simulink model "Kursovoy"  (Simulink 8.6)
settings: Solver=ode45  StartTime=0.0  StopTime=10  MaxStep=10e-6  RelTol=1e-3
values from neighbouring files (symbols this model uses):
  h_r = 0.9    [Drive1.m]    (also in Drive2.m; Drive3.m)
  i_r = 282.65    [Drive1.m]    (also in Drive2.m = 749.309; Drive3.m = 758.23)
  k_m = 0.704    [Drive1.m]    (also in Drive2.m = 0.694; Drive3.m = 0.744)
  k_p = 1.451E+4    (= 14510)    [Drive1.m]    (also in Drive2.m = 1621; Drive3.m = 1214)
  k_s = 6.41E+9    (= 6410000000)    [Drive1.m]    (also in Drive2.m = 1179000000; Drive3.m = 900400000)
  k_t = 1.787    [Drive1.m]    (also in Drive2.m = 1.208; Drive3.m = 3.846)
  Mdist_max = 1.326E+3    (= 1326)    [Drive1.m]    (also in Drive2.m = 15020; Drive3.m = 5965)
  Q_s = 0.991    [Drive1.m]    (also in Drive2.m = 0.412; Drive3.m = 0.252)
  T = 3.333E-6    (= 3.333e-06)    [Drive1.m]    (also in Drive2.m; Drive3.m)
  T1 = 0.219    [Drive1.m]    (also in Drive2.m = 0.415; Drive3.m = 0.289)
  T2 = 0.053    [Drive1.m]    (also in Drive2.m = 0.093; Drive3.m = 0.077)
  T5 = 7.559E-6    (= 7.559e-06)    [Drive1.m]    (also in Drive2.m = 1.323e-05; Drive3.m = 1.098e-05)
  Tau = 8.22E-4    (= 0.000822)    [Drive1.m]    (also in Drive2.m = 0.001429; Drive3.m = 0.001182)
  Te = 5.977E-3    (= 0.005977)    [Drive1.m]    (also in Drive2.m = 0.006546; Drive3.m = 0.004407)
  Tm = 0.098    [Drive1.m]    (also in Drive2.m = 0.03; Drive3.m = 0.025)
  w_max = 1.112    [Drive1.m]    (also in Drive2.m = 0.419; Drive3.m = 0.414)
  w_s = 1.122    [Drive1.m]    (also in Drive2.m = 1.017; Drive3.m = 1.646)
libraries: simulink x1
settings Model: Creator=divaise  LastModifiedBy=Admin
settings DebuggingCC: FcnCallInpInsideContextMsg=UseLocalSettings

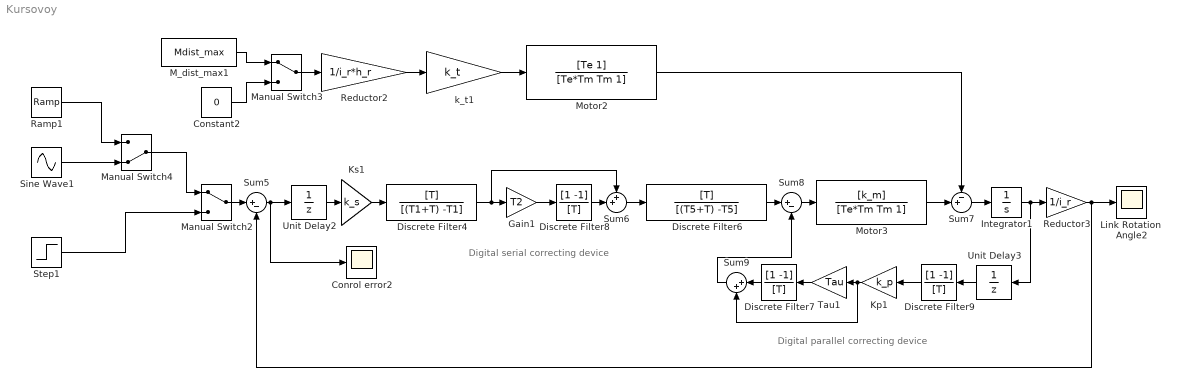
== system Kursovoy ==
  note: Digital serial correcting device
  note: Digital parallel correcting device
  Conrol error2 : Scope
  Constant2 : Constant  Value=0
  Discrete Filter4 : DiscreteFilter  Numerator=[T]  Denominator=[(T1+T) -T1]  SampleTime=T
  Discrete Filter6 : DiscreteFilter  Numerator=[T]  Denominator=[(T5+T) -T5]  SampleTime=T
  Discrete Filter7 : DiscreteFilter  Numerator=[1 -1]  Denominator=[T]  SampleTime=T
  Discrete Filter8 : DiscreteFilter  Numerator=[1 -1]  Denominator=[T]  SampleTime=T
  Discrete Filter9 : DiscreteFilter  Numerator=[1 -1]  Denominator=[T]  SampleTime=T
  Gain1 : Gain  Gain=T2
  Integrator1 : Integrator
  Kp1 : Gain  Gain=k_p
  Ks1 : Gain  Gain=k_s
  Link Rotation  Angle2 : Scope
  M_dist_max1 : Constant  Value=Mdist_max
  Manual Switch2 : ManualSwitch
  Manual Switch3 : ManualSwitch
  Manual Switch4 : ManualSwitch  CurrentSetting=0
  Motor2 : TransferFcn  Numerator=[Te 1]  Denominator=[Te*Tm Tm 1]
  Motor3 : TransferFcn  Numerator=[k_m]  Denominator=[Te*Tm Tm 1]
  Ramp1 : simulink/Sources/Ramp  slope=w_max  start=0  X0=0
  Reductor2 : Gain  Gain=1/i_r*h_r
  Reductor3 : Gain  Gain=1/i_r
  Sine Wave1 : Sin  Amplitude=Q_s  Frequency=w_s  SampleTime=0
  Step1 : Step  Time=0  SampleTime=0
  Sum5 : Sum  Inputs=|+-
  Sum6 : Sum  Inputs=++|
  Sum7 : Sum  Inputs=-+|
  Sum8 : Sum  Inputs=|+-
  Sum9 : Sum  Inputs=|++
  Tau1 : Gain  Gain=Tau
  Unit Delay2 : UnitDelay  SampleTime=T
  Unit Delay3 : UnitDelay  SampleTime=T
  k_t1 : Gain  Gain=k_t
  wires:
  Ramp1/1 -> Manual Switch4/1
  Sine Wave1/1 -> Manual Switch4/2
  Step1/1 -> Manual Switch2/2
  Manual Switch2/1 -> Sum5/1
  Reductor2/1 -> k_t1/1
  k_t1/1 -> Motor2/1
  Sum6/1 -> Discrete Filter6/1
  Motor3/1 -> Sum7/2
  Sum7/1 -> Integrator1/1
  Integrator1/1 -> Unit Delay3/1, Reductor3/1
  Reductor3/1 -> Link Rotation  Angle2/1, Sum5/2
  Kp1/1 -> Sum9/2, Tau1/1
  Motor2/1 -> Sum7/1
  Unit Delay2/1 -> Ks1/1
  Ks1/1 -> Discrete Filter4/1
  Discrete Filter4/1 -> Sum6/1, Gain1/1
  Discrete Filter6/1 -> Sum8/1
  Sum8/1 -> Motor3/1
  Sum9/1 -> Sum8/2
  Discrete Filter9/1 -> Kp1/1
  Tau1/1 -> Discrete Filter7/1
  Discrete Filter7/1 -> Sum9/1
  Discrete Filter8/1 -> Sum6/2
  Gain1/1 -> Discrete Filter8/1
  Sum5/1 -> Conrol error2/1, Unit Delay2/1
  Unit Delay3/1 -> Discrete Filter9/1
  Manual Switch4/1 -> Manual Switch2/1
  Manual Switch3/1 -> Reductor2/1
  M_dist_max1/1 -> Manual Switch3/1
  Constant2/1 -> Manual Switch3/2
